simulink model "Full_model_curve_fitted_spring_stiffness"  (R2018a)
settings: Solver=ode4  StartTime=0.0  StopTime=10.0  FixedStep=0.00000001  RelTol=1e-3
values from neighbouring files (symbols this model uses):
  bs = 2000    [suspensiondata.mat]
  bse = 3000    [suspensiondata.mat]
  Kse = 8000    [suspensiondata.mat]
  Kt = 125000    [suspensiondata.mat]
  Ms = 250    [suspensiondata.mat]
  Mse = 90    [suspensiondata.mat]
  Mu = 40    [suspensiondata.mat]
  Zr = 0.2    [suspensiondata.mat]
settings Model: Creator=Saurabh Suman  LastModifiedBy=Saurabh Suman

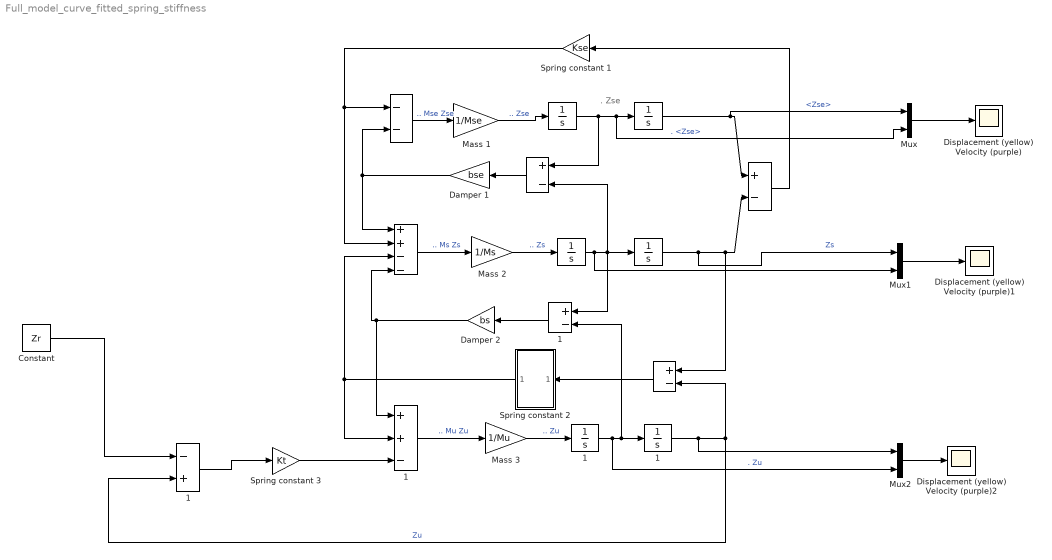
== system Full_model_curve_fitted_spring_stiffness ==
  note: .
      | Zse
  " " : Integrator
  "  " : Sum  Inputs=+-
  "     " : Integrator
  "      " : Sum  Inputs=++--
  "       " : Sum  Inputs=--
  "        " : Sum  Inputs=+-
  "         " : Integrator
  "          " : Integrator
  "             " : Sum  Inputs=+-
  "             1" : Sum  Inputs=+-
  "          1" : Integrator
  "         1" : Integrator
  "       1" : Sum  Inputs=-+
  "      1" : Sum  Inputs=++-
  Constant : Constant  Value=Zr
  Damper 1 : Gain  Gain=bse
  Damper 2 : Gain  Gain=bs
  Displacement (yellow) Velocity (purple) : Scope
  Displacement (yellow) Velocity (purple)1 : Scope
  Displacement (yellow) Velocity (purple)2 : Scope
  Mass 1 : Gain  Gain=1/Mse
  Mass 2 : Gain  Gain=1/Ms
  Mass 3 : Gain  Gain=1/Mu
  Mux : Mux  Inputs=2
  Mux1 : Mux  Inputs=2
  Mux2 : Mux  Inputs=2
  Spring constant 1 : Gain  Gain=Kse
  Spring constant 2 : Subsystem
  Spring constant 3 : Gain  Gain=Kt
  wires:
  Mux1/1 -> Displacement (yellow) Velocity (purple)1/1
  Mux/1 -> Displacement (yellow) Velocity (purple)/1
  "     "/1 -> "  "/1, Mux/1  "<Zse>"
  "       1"/1 -> Spring constant 3/1
  " "/1 -> "        "/1, "     "/1, Mux/2  ". <Zse>"
  Mass 1/1 -> " "/1  ".. Zse"
  Damper 1/1 -> "      "/1, "       "/2
  Damper 2/1 -> "      "/4, "      1"/1
  Spring constant 3/1 -> "      1"/3
  "          "/1 -> "  "/2, "             "/1, Mux1/1  "Zs"
  "      1"/1 -> Mass 3/1  ".. Mu Zu"
  "       "/1 -> Mass 1/1  ".. Mse Zse"
  Mass 3/1 -> "         1"/1  ".. Zu"
  "             1"/1 -> Damper 2/1
  "  "/1 -> Spring constant 1/1
  "         1"/1 -> "          1"/1, "             1"/2, Mux2/2  ". Zu"
  Mux2/1 -> Displacement (yellow) Velocity (purple)2/1
  Spring constant 2/1(Out1) -> "      "/3, "      1"/2
  "          1"/1 -> "             "/2, "       1"/2, Mux2/1  "Zu"
  Constant/1 -> "       1"/1
  Spring constant 1/1 -> "      "/2, "       "/1
  "             "/1 -> Spring constant 2/1(In3)
  "      "/1 -> Mass 2/1  ".. Ms Zs"
  Mass 2/1 -> "         "/1  ".. Zs"
  "         "/1 -> "        "/2, "          "/1, "             1"/1, Mux1/2
  "        "/1 -> Damper 1/1

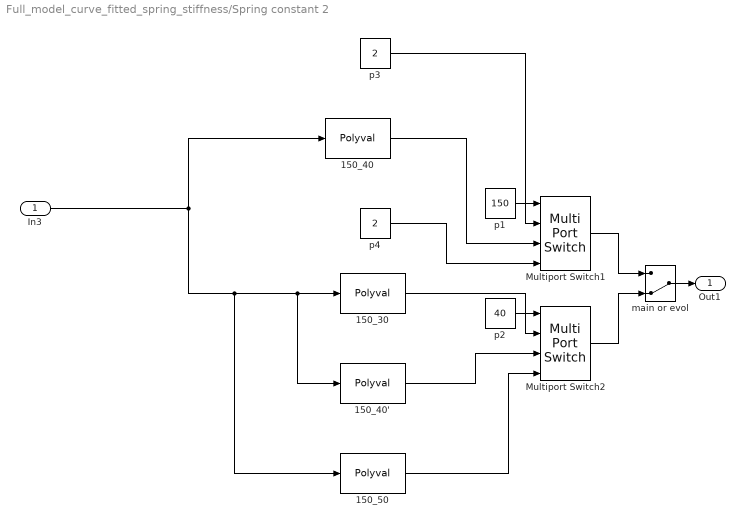
== system Full_model_curve_fitted_spring_stiffness/Spring constant 2 ==
  In3 : Inport
  150_30 : Polyval  Coefs=[ -5.674e+09*6, 1.562e+09*5, -1.485e+08*4, 6.452e+06*3, -1.365e+05*2, 3607 ]
  150_40 : Polyval  Coefs=[ -4.597e+09*6, 1.259e+09*5, -1.21e+08*4, 5.755e+06*3, -1.495e+05*2, 4352 ]
  150_40' : Polyval  Coefs=[ -4.597e+09*6, 1.259e+09*5, -1.21e+08*4, 5.755e+06*3, -1.495e+05*2, 4352 ]
  150_50 : Polyval  Coefs=[ -1.771e+09*6, 3.133e+08*5, -5.807e+06*4, -4.747e+05*3, 187.7*2, 3121 ]
  Multiport Switch1 : MultiPortSwitch  DataPortOrder=Specify indices  DataPortIndices={200,150,100}
  Multiport Switch2 : MultiPortSwitch  DataPortOrder=Specify indices  DataPortIndices={30,40,50}
  main or evol : ManualSwitch  CurrentSetting=0
  p1 : Constant  Value=150
  p2 : Constant  Value=40
  p3 : Constant  Value=2
  p4 : Constant  Value=2
  Out1 : Outport
  wires:
  main or evol/1 -> Out1/1
  p1/1 -> Multiport Switch1/1
  p2/1 -> Multiport Switch2/1
  Multiport Switch1/1 -> main or evol/1
  150_40'/1 -> Multiport Switch2/3
  Multiport Switch2/1 -> main or evol/2
  150_30/1 -> Multiport Switch2/2
  150_50/1 -> Multiport Switch2/4
  p4/1 -> Multiport Switch1/4
  150_40/1 -> Multiport Switch1/3
  p3/1 -> Multiport Switch1/2
  In3/1 -> 150_50/1, 150_40'/1, 150_30/1, 150_40/1
